simulink model "L6T1_SinglePhaseHBridgeCascaded"  (R2021a)
settings: Solver=VariableStepAuto  StartTime=0.0  StopTime=0.08  RelTol=1e-3
libraries: spsIGBTDiodeLib x8, spsDCVoltageSourceLib x2, spsTriangleGeneratorLib x2, spsCurrentMeasurementLib x1, spsSeriesRLCBranchLib x1, spsVoltageMeasurementLib x1, spspowerguiLib x1
settings Model: Creator=hp  LastModifiedBy=hp

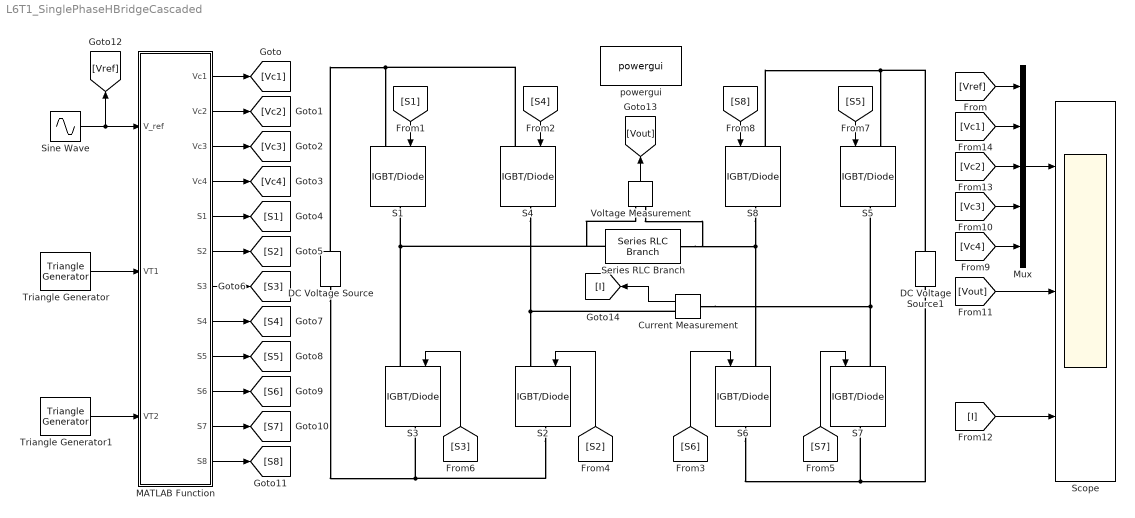
== system L6T1_SinglePhaseHBridgeCascaded ==
  Current Measurement : spsCurrentMeasurementLib/Current Measurement  PhasorSimulation=off  OutputType=Complex  PSBequivalent=0
  DC Voltage Source : spsDCVoltageSourceLib/DC Voltage Source  Amplitude=50  Measurements=None
  DC Voltage Source1 : spsDCVoltageSourceLib/DC Voltage Source  Amplitude=50  Measurements=None
  MATLAB Function : MATLAB Function  TreatAsAtomicUnit=on
  Mux : Mux  Inputs=5
  S{1..8} (8 alike) : spsIGBTDiodeLib/IGBT//Diode  Ron=1e-3  Rs=1e5  Cs=inf  Measurements=off
  Scope : Scope  NumInputPorts=3
  Series RLC Branch : spsSeriesRLCBranchLib/Series RLC Branch  LConnTagsString=__new0  RConnTagsString=__new0  BranchType=RL  Resistance=5  Inductance=100e-3  SetiL0=off  InitialCurrent=0  Capacitance=1e-6  Setx0=off  InitialVoltage=0  Measurements=None
  Sine Wave : Sin  Frequency=2*pi*50  SampleTime=0
  Triangle Generator : spsTriangleGeneratorLib/Triangle Generator  Freq=1000  Phase=0  Ts=0
  Triangle Generator1 : spsTriangleGeneratorLib/Triangle Generator  Freq=1000  Phase=180  Ts=0
  Voltage Measurement : spsVoltageMeasurementLib/Voltage Measurement  PhasorSimulation=off  OutputType=Complex  PSBequivalent=0
  powergui : spspowerguiLib/powergui  Priority=1  SimulationMode=Discrete  SampleTime=50e-6  frequency=60  Iterations=50  frequencyindice=0  Pbase=100e6  ErrMax=1e-4  UnitsV=kV  UnitsW=MW  buscounter=0  FunctionMessages=off  echomessages=off  EnableUseOfTLC=off  CurrentSourceSwitches=off  DisableSnubberDevices=off  DisableRonSwitches=off  DisableVfSwitches=off  DisplayEquations=off  AutomaticDiscreteSolvers=off  SolverType=Tustin/Backward Euler (TBE)  Interpol=off  ExternalGateDelay=off  methode=off  Ts=100  x0status=blocks  SPID=on  SwTol=0  HookPort=off  NonlinearTolerance=1e-4  nMaxIteration=100  ContinueOnMaxIteration=off  RestoreLinks=warning  ResistiveCurrentMeasurement=off  Frange=[0:2:500]  Ylog=off  Xlog=on  ShowGrid=off  save=off  variable=ZData  structure=0  ZoomFFT=off  StartTime=0.0  cycles=1  DisplayStyle=1  fundamental=60  FreqAxis=off  MaxFrequency=1000  frequencyindicesteady=1  RmsSteady=1  display=off
  wires:
  Sine Wave/1 -> [Vref], MATLAB Function/1(V_ref)
  Triangle Generator/1 -> MATLAB Function/2(VT1)
  Triangle Generator1/1 -> MATLAB Function/3(VT2)
  MATLAB Function/1(Vc1) -> [Vc1]
  MATLAB Function/2(Vc2) -> [Vc2]
  MATLAB Function/4(Vc4) -> [Vc4]
  MATLAB Function/3(Vc3) -> [Vc3]
  MATLAB Function/5(S1) -> [S1]
  MATLAB Function/6(S2) -> [S2]
  MATLAB Function/7(S3) -> [S3]
  MATLAB Function/8(S4) -> [S4]
  MATLAB Function/9(S5) -> [S5]
  MATLAB Function/11(S7) -> [S7]
  MATLAB Function/10(S6) -> [S6]
  MATLAB Function/12(S8) -> [S8]
  [Vref] -> Mux/1
  [S1] -> S1/1
  Mux/1 -> Scope/1
  [S4] -> S4/1
  [S8] -> S8/1
  [S5] -> S5/1
  [S3] -> S3/1
  [S2] -> S2/1
  [S6] -> S6/1
  [S7] -> S7/1
  [Vc3] -> Mux/4
  [Vc4] -> Mux/5
  [I] -> Scope/3
  [Vout] -> Scope/2
  [Vc2] -> Mux/3
  Voltage Measurement/1 -> [Vout]
  Current Measurement/1 -> [I]
  [Vc1] -> Mux/2
  connections:
  S3/LConn1 -- Voltage Measurement/LConn1 -- Series RLC Branch/LConn1 -- S1/RConn1
  S4/RConn1 -- Current Measurement/RConn1 -- S2/LConn1
  S4/LConn1 -- DC Voltage Source/RConn1 -- S1/LConn1
  S2/RConn1 -- DC Voltage Source/LConn1 -- S3/RConn1
  DC Voltage Source1/RConn1 -- S8/LConn1 -- S5/LConn1
  S6/RConn1 -- S7/RConn1 -- DC Voltage Source1/LConn1
  S7/LConn1 -- Current Measurement/LConn1 -- S5/RConn1
  S8/RConn1 -- Voltage Measurement/LConn2 -- Series RLC Branch/RConn1 -- S6/LConn1

== matlab function L6T1_SinglePhaseHBridgeCascaded/MATLAB Function ==
  data: V_ref input; Vc1 output; VT1 input; VT2 input; Vc2 output; Vc3 output; Vc4 output; S1 output; S2 output; S3 output; S4 output; S5 output; S6 output; S7 output; S8 output
function [Vc1,Vc2,Vc3,Vc4,S1,S2,S3,S4,S5,S6,S7,S8]= fcn(V_ref,VT1,VT2)
Vc2 = (VT1+1)*.25
Vc1 = ((VT1+3)*.25)
Vc3 = (VT2-1)*.25
Vc4 = ((VT2-3)*.25)
if V_ref>=0
    if V_ref>=0 && V_ref<0.5 
        if V_ref>=Vc2
            S1=1;    S2=1;    S3=0;    S4=0;
            S5=0;    S6=1;    S7=1;    S8=0;
        else
            S1=1;    S2=0;    S3=0;    S4=1;
            S5=1;    S6=0;    S7=0;    S8=1;
        end
    else V_ref>=0.5
        if V_ref>=Vc1
            S1=1;    S2=1;    S3=0;    S4=0;
            S5=1;    S6=1;    S7=0;    S8=0;
        else   
            S1=1;    S2=1;    S3=0;    S4=0;
            S5=1;    S6=0;    S7=0;    S8=1;
       end
    end
else
    if V_ref<0 && V_ref>=-0.5
        if V_ref<Vc3      
            S1=1;    S2=0;    S3=0;    S4=1;
            S5=0;    S6=0;    S7=1;    S8=1;
        else
            S1=1;    S2=0;    S3=0;    S4=1;
            S5=1;    S6=0;    S7=0;    S8=1;
        end
    else V_ref<=-0.5
        if V_ref<Vc4       
            S1=0;    S2=0;    S3=1;    S4=1;
            S5=0;    S6=0;    S7=1;    S8=1;
        else         
            S1=0;    S2=0;    S3=1;    S4=1;
            S5=1;    S6=0;    S7=0;    S8=1;
        end        
    end    
end
end
